simulink model "TestModel_3a"  (R2017b)
settings: Solver=VariableStepAuto  StartTime=0.0  StopTime=9000000  RelTol=1e-3
libraries: instrumentlib x2, svdutilitieslib x1
settings Model: Creator=koch  LastModifiedBy=koch

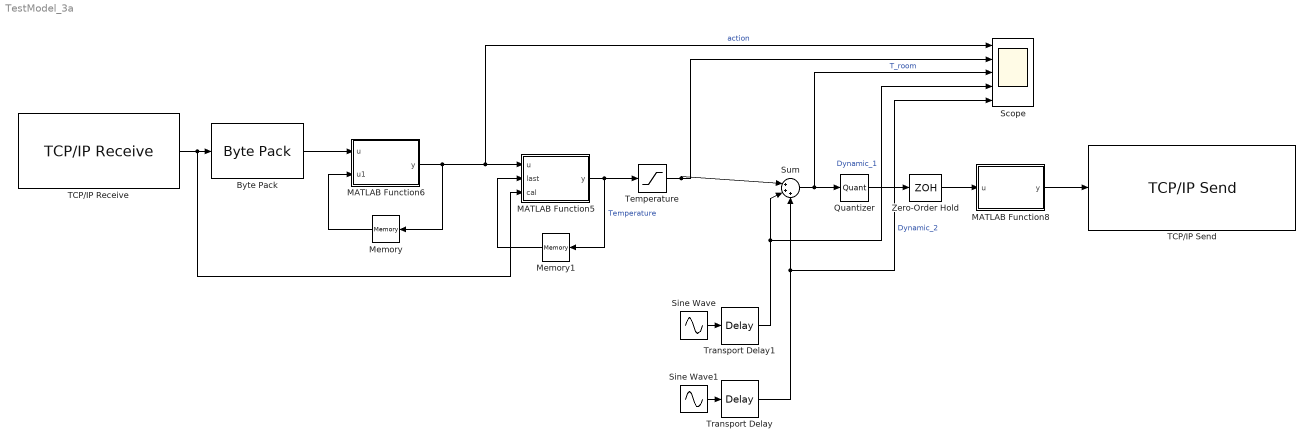
== system TestModel_3a ==
  Byte Pack : svdutilitieslib/Byte Pack  datatypes={'uint8'}  byteAlign=1  blockPlatform=arduinoert
      settings: SourceProductName=Simulink Support Package for Arduino Hardware  SourceProductBaseCode=ARDUINO
  MATLAB Function5 : MATLAB Function  TreatAsAtomicUnit=on
  MATLAB Function6 : MATLAB Function  TreatAsAtomicUnit=on
  MATLAB Function8 : MATLAB Function  TreatAsAtomicUnit=on
  Memory : Memory
  Memory1 : Memory  InitialCondition=24
  Quantizer : Quantizer  QuantizationInterval=0.1
  Scope : Scope  NumInputPorts=5
  Sine Wave : Sin  Amplitude=2  Frequency=0.00004  SampleTime=0
  Sine Wave1 : Sin  Amplitude=2  Frequency=0.0004  SampleTime=0
  Sum : Sum  Inputs=|+++
  TCP/IP Receive : instrumentlib/TCP//IP Receive  Host=localhost  Port=50000  DataSize=[1 1]  EnableBlockingMode=on  Timeout=10  SampleTime=200  DataType=uint8  ByteOrder=BigEndian
      settings: SourceProductName=Instrument Control Toolbox
  TCP/IP Send : instrumentlib/TCP//IP Send  Host=localhost  Port=50001  EnableBlockingMode=on  Timeout=10  ByteOrder=LittleEndian
      settings: SourceProductName=Instrument Control Toolbox
  Temperature : Saturate  UpperLimit=40  LowerLimit=15
  Transport Delay : TransportDelay  DelayTime=40000000
  Transport Delay1 : TransportDelay  DelayTime=20000000
  Zero-Order Hold : ZeroOrderHold  SampleTime=-1
  wires:
  Byte Pack/1 -> MATLAB Function6/1(u)
  Memory/1 -> MATLAB Function6/2(u1)
  TCP/IP Receive/1 -> MATLAB Function5/3(cal), Byte Pack/1
  Zero-Order Hold/1 -> MATLAB Function8/1(u)
  MATLAB Function8/1(y) -> TCP/IP Send/1
  Sum/1 -> Scope/3, Quantizer/1  "T_room"
  Sine Wave/1 -> Transport Delay1/1
  Transport Delay1/1 -> Scope/4, Sum/2  "Dynamic_1"
  Sine Wave1/1 -> Transport Delay/1
  Transport Delay/1 -> Scope/5, Sum/3  "Dynamic_2"
  Quantizer/1 -> Zero-Order Hold/1
  MATLAB Function6/1(y) -> Memory/1, Scope/1, MATLAB Function5/1(u)  "action"
  MATLAB Function5/1(y) -> Temperature/1, Memory1/1  "Temperature"
  Memory1/1 -> MATLAB Function5/2(last)
  Temperature/1 -> Sum/1, Scope/2

== matlab function TestModel_3a/MATLAB Function5 ==
  data: u input; y output; last input; cal input
function y = fcn(u,last,cal)

if cal > 0 
	k = 1;
else
    k = 0;
end


if u < 2 && k>0
    y = last;
    k = 0;
elseif 1 < u && u < 3 && k>0
    y = last -0.2;
    k = 0;
elseif 2 < u && k>0
    y = last+0.2;
    k = 0;
else
    y=last;
   
end
end

== matlab function TestModel_3a/MATLAB Function6 ==
  data: u input; y output; u1 input
function y  = fcn(u,u1)

u = double(u);
% zero is not a option so
if u > 0
    y = u;
else
    y = u1;
end

== matlab function TestModel_3a/MATLAB Function8 ==
  data: u input; y output
function y = fcn(u)


y = [u,4.5,4.6,4.7,4.8];
